simulink model "BER_calc_2_cycles"  (R2016b)
settings: Solver=VariableStepAuto  StartTime=0.0  StopTime=270  RelTol=1e-3
values from neighbouring files (symbols this model uses):
  det_data = [det_data_1(1:128) det_data_2(1+len:N)]    [BER_calc_script_2_cycles.m]
  true_data = sign(randn(1,N))>0    [BER_calc_script_2_cycles.m]
libraries: hdlsllib x3
settings Model: Creator=Arthur  LastModifiedBy=Arthur
settings OptimizationCC: DefaultParameterBehavior=Inlined

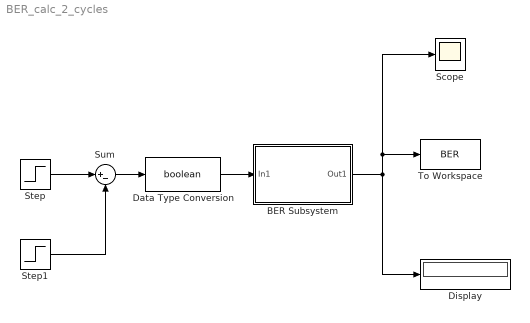
== system BER_calc_2_cycles ==
  BER Subsystem : Subsystem
  Data Type Conversion : DataTypeConversion  OutDataTypeStr=boolean
  Display : Display
  Scope : Scope
  Step : Step  Time=0  SampleTime=1
  Step1 : Step  SampleTime=1
  Sum : Sum  Inputs=|+-
  To Workspace : ToWorkspace  VariableName=BER  SampleTime=-1
  wires:
  Step1/1 -> Sum/2
  Step/1 -> Sum/1
  Sum/1 -> Data Type Conversion/1
  BER Subsystem/1(Out1) -> Scope/1, To Workspace/1, Display/1
  Data Type Conversion/1 -> BER Subsystem/1(In1)

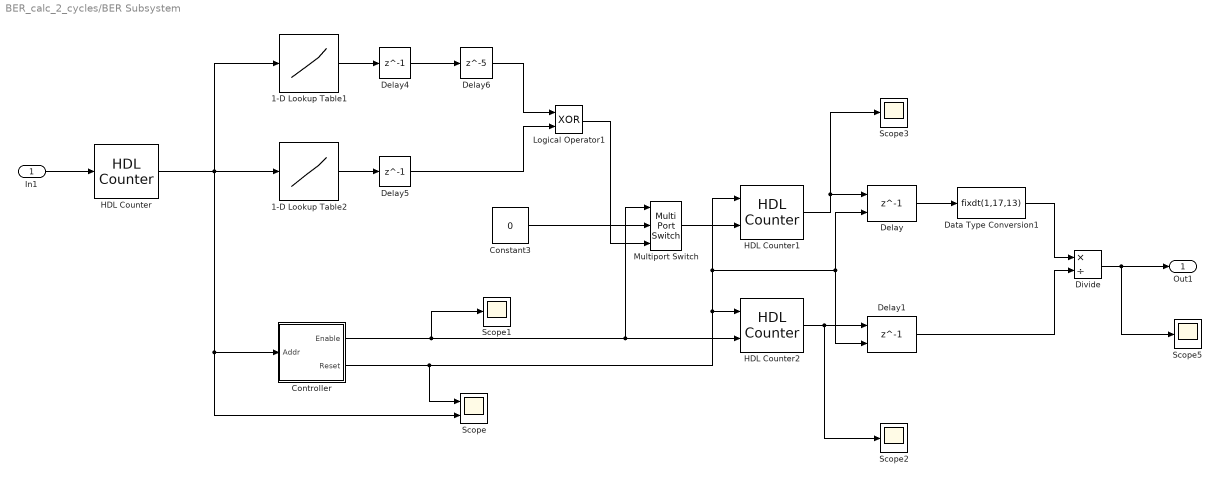
== system BER_calc_2_cycles/BER Subsystem ==
  In1 : Inport
  1-D Lookup Table1 : Lookup_n-D  NumberOfTableDimensions=1  BreakpointsForDimension1=[0:255]  BreakpointsForDimension1FirstPoint=10  BreakpointsForDimension2FirstPoint=10  BreakpointsForDimension1Spacing=12  BreakpointsForDimension2Spacing=12  IndexSearchMethod=Evenly spaced points  Table=true_data*1  InterpMethod=Flat  DiagnosticForOutOfRangeInput=Error  InternalRulePriority=Speed  RndMeth=Simplest  InputSameDT=on
  1-D Lookup Table2 : Lookup_n-D  NumberOfTableDimensions=1  BreakpointsForDimension1=[0:255]  BreakpointsForDimension1FirstPoint=10  BreakpointsForDimension2FirstPoint=10  BreakpointsForDimension1Spacing=12  BreakpointsForDimension2Spacing=12  IndexSearchMethod=Evenly spaced points  Table=det_data*1  InterpMethod=Flat  DiagnosticForOutOfRangeInput=Error  InternalRulePriority=Speed  RndMeth=Simplest  InputSameDT=on
  Constant3 : Constant  Value=0  VectorParams1D=off  OutDataTypeStr=boolean  SampleTime=-1
  Controller : Subsystem
  Data Type Conversion1 : DataTypeConversion  OutDataTypeStr=fixdt(1,17,13)
  Delay : Delay  DelayLength=1  InitialCondition=0  ExternalReset=Rising  UseCircularBuffer=on
      settings: InputPortMap=u0,r5
  Delay1 : Delay  DelayLength=1  InitialCondition=0  ExternalReset=Rising  UseCircularBuffer=on
      settings: InputPortMap=u0,r5
  Delay4 : Delay  DelayLength=1
  Delay5 : Delay  DelayLength=1
  Delay6 : Delay  DelayLength=5
  Divide : Product  Inputs=*/  OutDataTypeStr=fixdt(1,17,13)
  HDL Counter : hdlsllib/HDL Operations/HDL Counter  CountType=Count limited  CountInit=0  CountStep=1  CountMax=255  CountFromType=Initial value  CountFrom=0  CountResetPort=on  CountLoadPort=off  CountEnbPort=off  CountDirPort=off  CountDataType=Signed  CountWordLen=17  CountFracLen=0  CountSampTime=1
  HDL Counter1 : hdlsllib/HDL Operations/HDL Counter  CountType=Free running  CountInit=0  CountStep=1  CountMax=25  CountFromType=Specify  CountFrom=0  CountResetPort=on  CountLoadPort=off  CountEnbPort=on  CountDirPort=off  CountDataType=Signed  CountWordLen=17  CountFracLen=0  CountSampTime=1
  HDL Counter2 : hdlsllib/HDL Operations/HDL Counter  CountType=Count limited  CountInit=1  CountStep=1  CountMax=128  CountFromType=Specify  CountFrom=1  CountResetPort=on  CountLoadPort=off  CountEnbPort=on  CountDirPort=off  CountDataType=Signed  CountWordLen=17  CountFracLen=0  CountSampTime=1
  Logical Operator1 : Logic  Operator=XOR  AllPortsSameDT=off  OutDataTypeStr=boolean
  Multiport Switch : MultiPortSwitch  DataPortOrder=Zero-based contiguous  Inputs=2
  Scope : Scope  NumInputPorts=2
  Scope{1..3,5} (4 alike) : Scope
  Out1 : Outport
  wires:
  Delay4/1 -> Delay6/1
  Delay6/1 -> Logical Operator1/1
  Delay5/1 -> Logical Operator1/2
  Controller/1(Enable) -> Scope1/1, Multiport Switch/1, HDL Counter2/2
  Constant3/1 -> Multiport Switch/2
  Divide/1 -> Scope5/1, Out1/1
  HDL Counter2/1 -> Delay1/1, Scope2/1
  HDL Counter1/1 -> Scope3/1, Delay/1
  Delay1/1 -> Divide/2
  Data Type Conversion1/1 -> Divide/1
  Delay/1 -> Data Type Conversion1/1
  HDL Counter/1 -> 1-D Lookup Table2/1, 1-D Lookup Table1/1, Scope/2, Controller/1(Addr)
  Controller/2(Reset) -> Scope/1, Delay1/2, Delay/2, HDL Counter1/1, HDL Counter2/1
  Multiport Switch/1 -> HDL Counter1/2
  In1/1 -> HDL Counter/1
  1-D Lookup Table2/1 -> Delay5/1
  1-D Lookup Table1/1 -> Delay4/1
  Logical Operator1/1 -> Multiport Switch/3

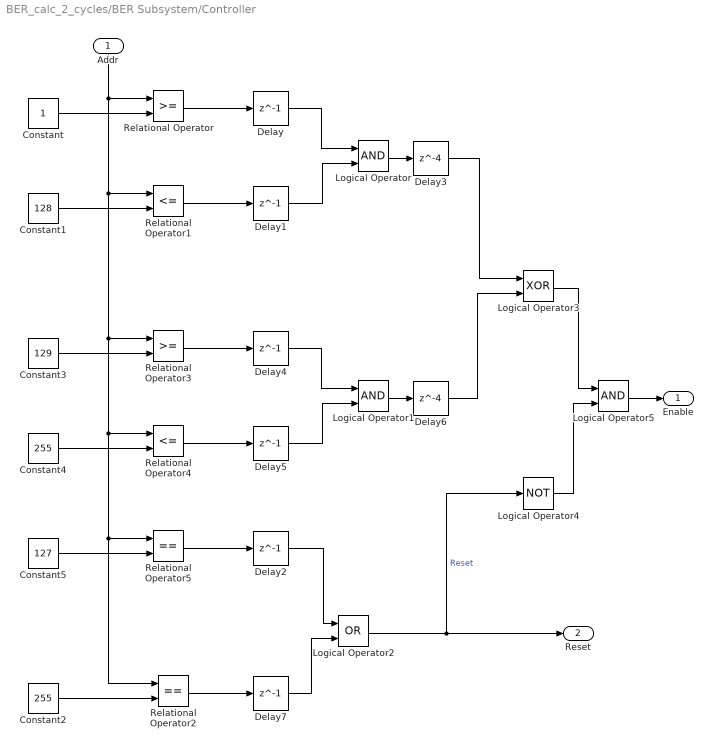
== system BER_calc_2_cycles/BER Subsystem/Controller ==
  Addr : Inport
  Constant : Constant  OutDataTypeStr=fixdt(0,10,0)
  Constant1 : Constant  Value=128  OutDataTypeStr=fixdt(0,10,0)
  Constant2 : Constant  Value=255  OutDataTypeStr=fixdt(0,10,0)
  Constant3 : Constant  Value=129  OutDataTypeStr=fixdt(0,10,0)
  Constant4 : Constant  Value=255  OutDataTypeStr=fixdt(0,10,0)
  Constant5 : Constant  Value=127  OutDataTypeStr=fixdt(0,10,0)
  Delay{,1..2,4..5,7} (6 alike) : Delay  DelayLength=1
  Delay3 : Delay  DelayLength=4
  Delay6 : Delay  DelayLength=4
  Logical Operator : Logic  AllPortsSameDT=off  OutDataTypeStr=boolean
  Logical Operator1 : Logic  AllPortsSameDT=off  OutDataTypeStr=boolean
  Logical Operator2 : Logic  Operator=OR  AllPortsSameDT=off  OutDataTypeStr=boolean
  Logical Operator3 : Logic  Operator=XOR  AllPortsSameDT=off  OutDataTypeStr=boolean
  Logical Operator4 : Logic  Operator=NOT  AllPortsSameDT=off  OutDataTypeStr=boolean
  Logical Operator5 : Logic  AllPortsSameDT=off  OutDataTypeStr=boolean
  Relational Operator : RelationalOperator  OutDataTypeStr=boolean  RndMeth=Simplest
  Relational Operator1 : RelationalOperator  Operator=<=  OutDataTypeStr=boolean  RndMeth=Nearest
  Relational Operator2 : RelationalOperator  Operator===  OutDataTypeStr=boolean  RndMeth=Simplest
  Relational Operator3 : RelationalOperator  OutDataTypeStr=boolean  RndMeth=Simplest
  Relational Operator4 : RelationalOperator  Operator=<=  OutDataTypeStr=boolean  RndMeth=Nearest
  Relational Operator5 : RelationalOperator  Operator===  OutDataTypeStr=boolean  RndMeth=Simplest
  Enable : Outport
  Reset : Outport  Port=2
  wires:
  Constant/1 -> Relational Operator/2
  Constant1/1 -> Relational Operator1/2
  Logical Operator/1 -> Delay3/1
  Delay/1 -> Logical Operator/1
  Relational Operator/1 -> Delay/1
  Relational Operator1/1 -> Delay1/1
  Delay1/1 -> Logical Operator/2
  Constant3/1 -> Relational Operator3/2
  Constant4/1 -> Relational Operator4/2
  Logical Operator1/1 -> Delay6/1
  Delay4/1 -> Logical Operator1/1
  Relational Operator3/1 -> Delay4/1
  Relational Operator4/1 -> Delay5/1
  Delay5/1 -> Logical Operator1/2
  Constant5/1 -> Relational Operator5/2
  Relational Operator5/1 -> Delay2/1
  Addr/1 -> Relational Operator3/1, Relational Operator4/1, Relational Operator5/1, Relational Operator2/1, Relational Operator1/1, Relational Operator/1
  Constant2/1 -> Relational Operator2/2
  Relational Operator2/1 -> Delay7/1
  Delay7/1 -> Logical Operator2/2
  Delay2/1 -> Logical Operator2/1
  Logical Operator2/1 -> Logical Operator4/1, Reset/1  "Reset"
  Delay6/1 -> Logical Operator3/2
  Delay3/1 -> Logical Operator3/1
  Logical Operator5/1 -> Enable/1
  Logical Operator3/1 -> Logical Operator5/1
  Logical Operator4/1 -> Logical Operator5/2
